simulink model "SimFinal"  (R2023a)
settings: Solver=VariableStepAuto  StartTime=0.0  StopTime=4.88  RelTol=1e-3
settings Model: Creator=cesar.cruz  LastModifiedBy=cesar.cruz
settings DataIOCC: ReturnWorkspaceOutputs=off

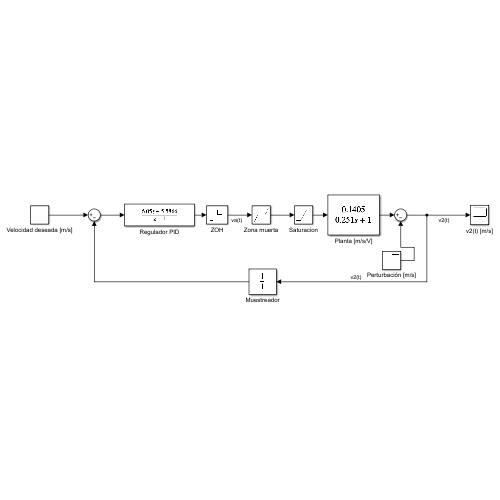
[thumbnail: Simulink's stored preview of the top-level diagram]
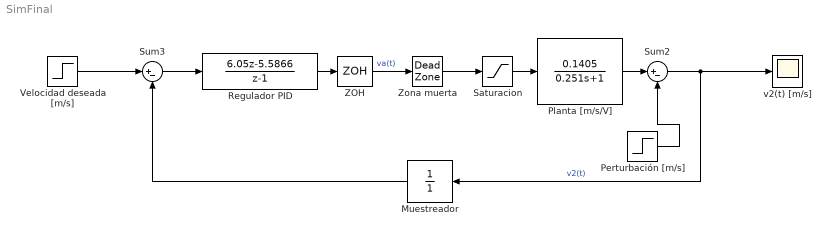
== system SimFinal ==
  Muestreador : TransferFcn  Numerator=1  Denominator=1
  Perturbación [m/s] : Step  Time=1.62  After=0.2  SampleTime=0
  Planta [m/s/V] : TransferFcn  Numerator=[0.1405]  Denominator=[0.251 1]
  Regulador PID : DiscreteTransferFcn  Numerator=[6.05,-5.5866]  Denominator=[1 -1]  SampleTime=20e-3
  Saturacion : Saturate  UpperLimit=9.8  LowerLimit=-9.8
  Sum2 : Sum  Inputs=|+-
  Sum3 : Sum  Inputs=|+-
  Velocidad deseada [m/s] : Step  Time=0  After=-1  SampleTime=0
  ZOH : ZeroOrderHold  SampleTime=20e-3
  Zona muerta : DeadZone
  v2(t) [m/s] : Scope
  wires:
  Saturacion/1 -> Planta [m/s/V]/1
  Sum2/1 -> v2(t) [m/s]/1, Muestreador/1  "v2(t)"
  Velocidad deseada [m/s]/1 -> Sum3/1
  Muestreador/1 -> Sum3/2
  Planta [m/s/V]/1 -> Sum2/1
  Sum3/1 -> Regulador PID/1
  Regulador PID/1 -> ZOH/1
  Perturbación [m/s]/1 -> Sum2/2
  ZOH/1 -> Zona muerta/1  "va(t)"
  Zona muerta/1 -> Saturacion/1
